simulink model "controladores_LAB4"  (R2023b)
settings: Solver=ode23t  StartTime=0.0  StopTime=110  RelTol=1e-3
values from neighbouring files (symbols this model uses):
  Blo = 8.18575752786119e-06    (= 8.18575752786e-06)    [modeloMATEMATICOFINAL.m]
  Bmo = 2.02156082362446e-07    (= 2.02156082362e-07)    [modeloMATEMATICOFINAL.m]
  CL = double(subs(C_par))    [modeloMATEMATICOFINAL.m]
  DL = double(subs(D_par))    [modeloMATEMATICOFINAL.m]
  do = 0.06862-0.021    (= 0.04762)    [modeloMATEMATICOFINAL.m]
  GL = sysd.a    [modeloMATEMATICOFINAL.m]
  go = 9.81    [modeloMATEMATICOFINAL.m]
  HL = sysd.b    [modeloMATEMATICOFINAL.m]
  Jlo = 0.00100697016255642    (= 0.00100697016256)    [modeloMATEMATICOFINAL.m]
  Jmo = 2.08549279330578e-07    (= 2.08549279331e-07)    [modeloMATEMATICOFINAL.m]
  Kio = 0.00119530882984502    (= 0.00119530882985)    [modeloMATEMATICOFINAL.m]
  Kvo = 0.0035694528924319    (= 0.00356945289243)    [modeloMATEMATICOFINAL.m]
  Lo = 0.667669785204658    (= 0.667669785205)    [modeloMATEMATICOFINAL.m]
  mo = 0.17244    [modeloMATEMATICOFINAL.m]
  no = 120    [modeloMATEMATICOFINAL.m]
  Ro = 5.15610211779038    (= 5.15610211779)    [modeloMATEMATICOFINAL.m]
  Tm = 0.03    [modeloMATEMATICOFINAL.m]
  Vin0 = Ro*X10    (= 0)    [modeloMATEMATICOFINAL.m]
  X10 = 0    [modeloMATEMATICOFINAL.m]
  X20 = 0    [modeloMATEMATICOFINAL.m]
  X30 = 0    [modeloMATEMATICOFINAL.m]
libraries: simulink x8, cstblocks x8
settings Model: Creator=hubertdelgado  LastModifiedBy=automatizacion
settings DebuggingCC: UnconnectedInputMsg=warning  UnconnectedOutputMsg=warning  UnconnectedLineMsg=warning
settings ModelReferenceCC: EnableRefExpFcnMdlSchedulingChecks=on
settings RTWCC: DLArmComputeVersion=19.05

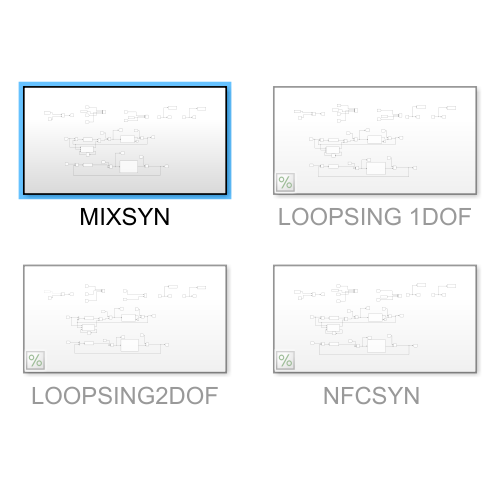
[thumbnail: Simulink's stored preview of the top-level diagram]
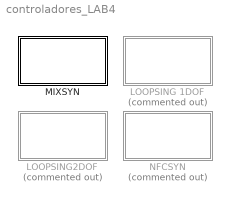
== system controladores_LAB4 ==
  LOOPSING 1DOF : Subsystem  Commented=on
  LOOPSING2DOF : Subsystem  Commented=on
  MIXSYN : Subsystem
  "NFCSYN " : Subsystem  Commented=on

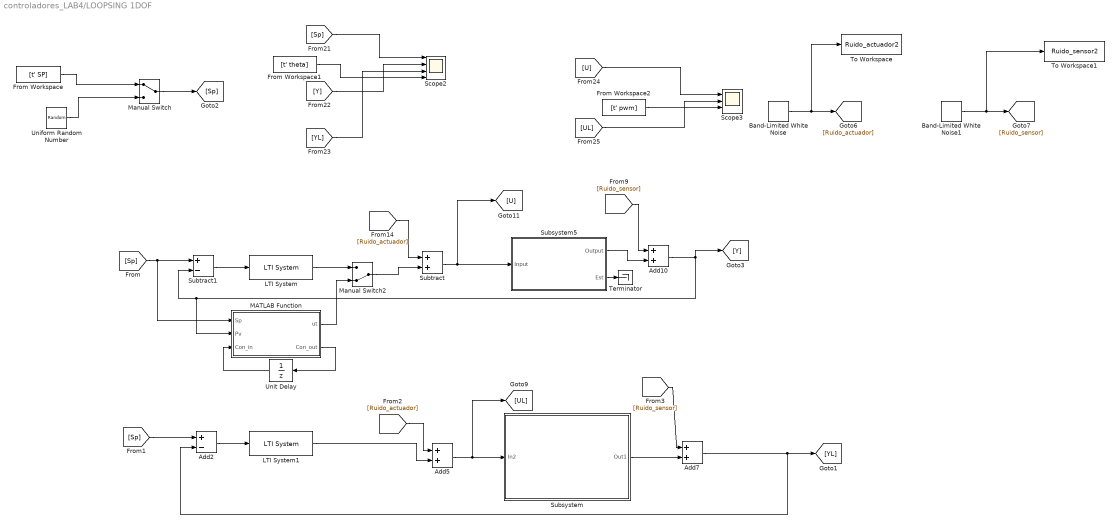
== system controladores_LAB4/LOOPSING 1DOF ==
  Add10 : Sum
  Add2 : Sum  Inputs=+-
  Add5 : Sum
  Add7 : Sum
  Band-Limited White Noise : simulink/Sources/Band-Limited White Noise  Cov=[1e-8]  Ts=0.001  seed=[23341]
  Band-Limited White Noise1 : simulink/Sources/Band-Limited White Noise  Cov=[1e-8]  Ts=0.001  seed=[23341]
  From Workspace : FromWorkspace  VariableName=[t' SP]
  From Workspace1 : FromWorkspace  VariableName=[t' theta]
  From Workspace2 : FromWorkspace  VariableName=[t' pwm]
  LTI System : cstblocks/LTI System  sys=Kred  IC=[]  PadeOrder=0
  LTI System1 : cstblocks/LTI System  sys=Kred  IC=[]  PadeOrder=0
  MATLAB Function : MATLAB Function  TreatAsAtomicUnit=on
  Manual Switch : ManualSwitch
  Manual Switch2 : ManualSwitch  CurrentSetting=0
  Scope2 : Scope  NumInputPorts=4
  Scope3 : Scope  NumInputPorts=3
  Subsystem : Subsystem
  Subsystem5 : Subsystem
  Subtract : Sum
  Subtract1 : Sum  Inputs=+-
  Terminator : Terminator
  To Workspace : ToWorkspace  VariableName=Ruido_actuador2  SampleTime=-1
  To Workspace1 : ToWorkspace  VariableName=Ruido_sensor2  SampleTime=-1
  Uniform Random Number : UniformRandomNumber  Minimum=-70*(pi/180)  Maximum=70*(pi/180)  SampleTime=10
  Unit Delay : UnitDelay  InitialCondition=zeros(4,1)  SampleTime=Tm  HasFrameUpgradeWarning=on
  wires:
  Add5/1 -> [UL], Subsystem/1(In2)
  [Ruido_sensor] -> Add10/1
  [Ruido_actuador] -> Subtract/1
  [Ruido_sensor] -> Add7/1
  Add7/1 -> Add2/2, [YL]
  Subsystem5/1(Output) -> Add10/2
  Subtract/1 -> Subsystem5/1(Input), [U]
  Band-Limited White Noise/1 -> To Workspace/1, [Ruido_actuador]
  Band-Limited White Noise1/1 -> To Workspace1/1, [Ruido_sensor]
  [Ruido_actuador] -> Add5/1
  Add10/1 -> [Y], MATLAB Function/2(Pv), Subtract1/2
  Add2/1 -> LTI System1/1
  [Sp] -> Add2/1
  Subsystem5/2(Est) -> Terminator/1
  Subtract1/1 -> LTI System/1
  LTI System/1 -> Manual Switch2/1
  Manual Switch2/1 -> Subtract/2
  [Sp] -> MATLAB Function/1(Sp), Subtract1/1
  Subsystem/1(Out1) -> Add7/2
  LTI System1/1 -> Add5/2
  Unit Delay/1 -> MATLAB Function/3(Con_in)
  MATLAB Function/1(ut) -> Manual Switch2/2
  MATLAB Function/2(Con_out) -> Unit Delay/1
  [YL] -> Scope2/3
  [Sp] -> Scope2/1
  Uniform Random Number/1 -> Manual Switch/2
  [U] -> Scope3/1
  [UL] -> Scope3/2
  From Workspace/1 -> Manual Switch/1
  Manual Switch/1 -> [Sp]
  [Y] -> Scope2/2
  From Workspace1/1 -> Scope2/4
  From Workspace2/1 -> Scope3/3

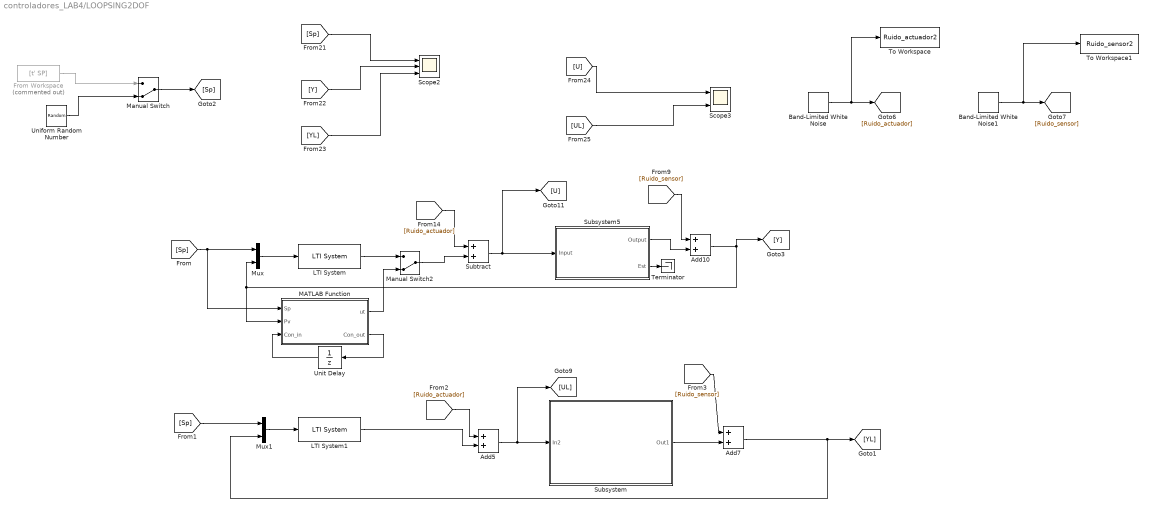
== system controladores_LAB4/LOOPSING2DOF ==
  Add10 : Sum
  Add5 : Sum
  Add7 : Sum
  Band-Limited White Noise : simulink/Sources/Band-Limited White Noise  Cov=[1e-8]  Ts=0.001  seed=[23341]
  Band-Limited White Noise1 : simulink/Sources/Band-Limited White Noise  Cov=[1e-8]  Ts=0.001  seed=[23341]
  From Workspace : FromWorkspace  Commented=on  VariableName=[t' SP]
  LTI System : cstblocks/LTI System  sys=Kred2dof  IC=[]  PadeOrder=0
  LTI System1 : cstblocks/LTI System  sys=Kred2dof  IC=[]  PadeOrder=0
  MATLAB Function : MATLAB Function  TreatAsAtomicUnit=on
  Manual Switch : ManualSwitch  CurrentSetting=0
  Manual Switch2 : ManualSwitch  CurrentSetting=0
  Mux : Mux  Inputs=2
  Mux1 : Mux  Inputs=2
  Scope2 : Scope  NumInputPorts=3
  Scope3 : Scope  NumInputPorts=2
  Subsystem : Subsystem
  Subsystem5 : Subsystem
  Subtract : Sum
  Terminator : Terminator
  To Workspace : ToWorkspace  VariableName=Ruido_actuador2  SampleTime=-1
  To Workspace1 : ToWorkspace  VariableName=Ruido_sensor2  SampleTime=-1
  Uniform Random Number : UniformRandomNumber  Minimum=-70*(pi/180)  Maximum=70*(pi/180)  SampleTime=10
  Unit Delay : UnitDelay  InitialCondition=zeros(5,1)  SampleTime=Tm  HasFrameUpgradeWarning=on
  wires:
  MATLAB Function/1(ut) -> Manual Switch2/2
  Unit Delay/1 -> MATLAB Function/3(Con_in)
  LTI System1/1 -> Add5/2
  Subsystem/1(Out1) -> Add7/2
  [Sp] -> Mux/1, MATLAB Function/1(Sp)
  Manual Switch2/1 -> Subtract/2
  LTI System/1 -> Manual Switch2/1
  Subsystem5/2(Est) -> Terminator/1
  [Sp] -> Mux1/1
  Mux1/1 -> LTI System1/1
  Add10/1 -> Mux/2, MATLAB Function/2(Pv), [Y]
  [Ruido_actuador] -> Add5/1
  Band-Limited White Noise1/1 -> [Ruido_sensor], To Workspace1/1
  Band-Limited White Noise/1 -> [Ruido_actuador], To Workspace/1
  Subtract/1 -> [U], Subsystem5/1(Input)
  Subsystem5/1(Output) -> Add10/2
  Add7/1 -> Mux1/2, [YL]
  [Ruido_sensor] -> Add7/1
  [Ruido_actuador] -> Subtract/1
  [Ruido_sensor] -> Add10/1
  Add5/1 -> Subsystem/1(In2), [UL]
  MATLAB Function/2(Con_out) -> Unit Delay/1
  Mux/1 -> LTI System/1
  [Y] -> Scope2/2
  [U] -> Scope3/1
  From Workspace/1 -> Manual Switch/1
  Uniform Random Number/1 -> Manual Switch/2
  [UL] -> Scope3/2
  [YL] -> Scope2/3
  [Sp] -> Scope2/1
  Manual Switch/1 -> [Sp]

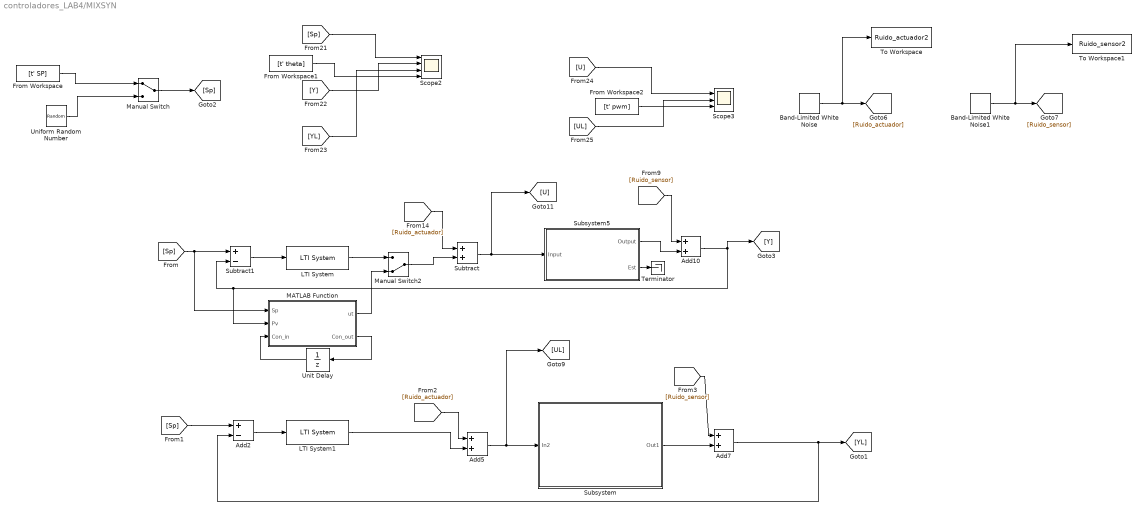
== system controladores_LAB4/MIXSYN ==
  Add10 : Sum
  Add2 : Sum  Inputs=+-
  Add5 : Sum
  Add7 : Sum
  Band-Limited White Noise : simulink/Sources/Band-Limited White Noise  Cov=[1e-8]  Ts=0.001  seed=[23341]
  Band-Limited White Noise1 : simulink/Sources/Band-Limited White Noise  Cov=[1e-8]  Ts=0.001  seed=[23341]
  From Workspace : FromWorkspace  VariableName=[t' SP]
  From Workspace1 : FromWorkspace  VariableName=[t' theta]
  From Workspace2 : FromWorkspace  VariableName=[t' pwm]
  LTI System : cstblocks/LTI System  sys=Kred  IC=[]  PadeOrder=0
  LTI System1 : cstblocks/LTI System  sys=Kred  IC=[]  PadeOrder=0
  MATLAB Function : MATLAB Function  TreatAsAtomicUnit=on
  Manual Switch : ManualSwitch
  Manual Switch2 : ManualSwitch  CurrentSetting=0
  Scope2 : Scope  NumInputPorts=4
  Scope3 : Scope  NumInputPorts=3
  Subsystem : Subsystem
  Subsystem5 : Subsystem
  Subtract : Sum
  Subtract1 : Sum  Inputs=+-
  Terminator : Terminator
  To Workspace : ToWorkspace  VariableName=Ruido_actuador2  SampleTime=-1
  To Workspace1 : ToWorkspace  VariableName=Ruido_sensor2  SampleTime=-1
  Uniform Random Number : UniformRandomNumber  Minimum=-70*(pi/180)  Maximum=70*(pi/180)  SampleTime=10
  Unit Delay : UnitDelay  InitialCondition=zeros(5,1)  SampleTime=Tm  HasFrameUpgradeWarning=on
  wires:
  [Sp] -> Scope2/1
  Add5/1 -> [UL], Subsystem/1(In2)
  [Ruido_sensor] -> Add10/1
  [Ruido_actuador] -> Subtract/1
  [Ruido_sensor] -> Add7/1
  Add7/1 -> Add2/2, [YL]
  [Y] -> Scope2/2
  Subsystem5/1(Output) -> Add10/2
  [YL] -> Scope2/3
  Subtract/1 -> Subsystem5/1(Input), [U]
  Band-Limited White Noise/1 -> To Workspace/1, [Ruido_actuador]
  Band-Limited White Noise1/1 -> To Workspace1/1, [Ruido_sensor]
  Manual Switch/1 -> [Sp]
  [UL] -> Scope3/2
  From Workspace/1 -> Manual Switch/1
  [U] -> Scope3/1
  Uniform Random Number/1 -> Manual Switch/2
  [Ruido_actuador] -> Add5/1
  Add10/1 -> [Y], MATLAB Function/2(Pv), Subtract1/2
  Add2/1 -> LTI System1/1
  [Sp] -> Add2/1
  Subsystem5/2(Est) -> Terminator/1
  Subtract1/1 -> LTI System/1
  LTI System/1 -> Manual Switch2/1
  Manual Switch2/1 -> Subtract/2
  [Sp] -> MATLAB Function/1(Sp), Subtract1/1
  Subsystem/1(Out1) -> Add7/2
  LTI System1/1 -> Add5/2
  Unit Delay/1 -> MATLAB Function/3(Con_in)
  MATLAB Function/1(ut) -> Manual Switch2/2
  MATLAB Function/2(Con_out) -> Unit Delay/1
  From Workspace1/1 -> Scope2/4
  From Workspace2/1 -> Scope3/3

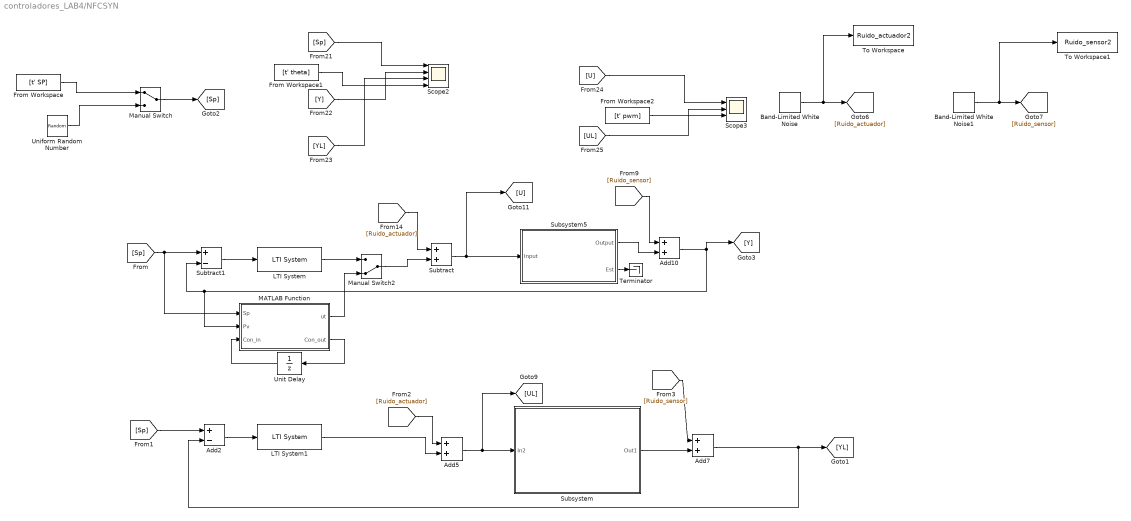
== system controladores_LAB4/NFCSYN  ==
  Add10 : Sum
  Add2 : Sum  Inputs=+-
  Add5 : Sum
  Add7 : Sum
  Band-Limited White Noise : simulink/Sources/Band-Limited White Noise  Cov=[1e-8]  Ts=0.001  seed=[23341]
  Band-Limited White Noise1 : simulink/Sources/Band-Limited White Noise  Cov=[1e-8]  Ts=0.001  seed=[23341]
  From Workspace : FromWorkspace  VariableName=[t' SP]
  From Workspace1 : FromWorkspace  VariableName=[t' theta]
  From Workspace2 : FromWorkspace  VariableName=[t' pwm]
  LTI System : cstblocks/LTI System  sys=Kred  IC=[]  PadeOrder=0
  LTI System1 : cstblocks/LTI System  sys=Kred  IC=[]  PadeOrder=0
  MATLAB Function : MATLAB Function  TreatAsAtomicUnit=on
  Manual Switch : ManualSwitch
  Manual Switch2 : ManualSwitch  CurrentSetting=0
  Scope2 : Scope  NumInputPorts=4
  Scope3 : Scope  NumInputPorts=3
  Subsystem : Subsystem
  Subsystem5 : Subsystem
  Subtract : Sum
  Subtract1 : Sum  Inputs=+-
  Terminator : Terminator
  To Workspace : ToWorkspace  VariableName=Ruido_actuador2  SampleTime=-1
  To Workspace1 : ToWorkspace  VariableName=Ruido_sensor2  SampleTime=-1
  Uniform Random Number : UniformRandomNumber  Minimum=-70*(pi/180)  Maximum=70*(pi/180)  SampleTime=10
  Unit Delay : UnitDelay  InitialCondition=zeros(4,1)  SampleTime=Tm  HasFrameUpgradeWarning=on
  wires:
  Add5/1 -> [UL], Subsystem/1(In2)
  [Ruido_sensor] -> Add10/1
  [Ruido_actuador] -> Subtract/1
  [Ruido_sensor] -> Add7/1
  Add7/1 -> Add2/2, [YL]
  Subsystem5/1(Output) -> Add10/2
  Subtract/1 -> Subsystem5/1(Input), [U]
  Band-Limited White Noise/1 -> To Workspace/1, [Ruido_actuador]
  Band-Limited White Noise1/1 -> To Workspace1/1, [Ruido_sensor]
  [Ruido_actuador] -> Add5/1
  Add10/1 -> [Y], MATLAB Function/2(Pv), Subtract1/2
  Add2/1 -> LTI System1/1
  [Sp] -> Add2/1
  Subsystem5/2(Est) -> Terminator/1
  Subtract1/1 -> LTI System/1
  LTI System/1 -> Manual Switch2/1
  Manual Switch2/1 -> Subtract/2
  [Sp] -> MATLAB Function/1(Sp), Subtract1/1
  Subsystem/1(Out1) -> Add7/2
  LTI System1/1 -> Add5/2
  Unit Delay/1 -> MATLAB Function/3(Con_in)
  MATLAB Function/1(ut) -> Manual Switch2/2
  MATLAB Function/2(Con_out) -> Unit Delay/1
  From Workspace1/1 -> Scope2/4
  [Y] -> Scope2/2
  [U] -> Scope3/1
  From Workspace/1 -> Manual Switch/1
  Uniform Random Number/1 -> Manual Switch/2
  [UL] -> Scope3/2
  [YL] -> Scope2/3
  [Sp] -> Scope2/1
  Manual Switch/1 -> [Sp]
  From Workspace2/1 -> Scope3/3

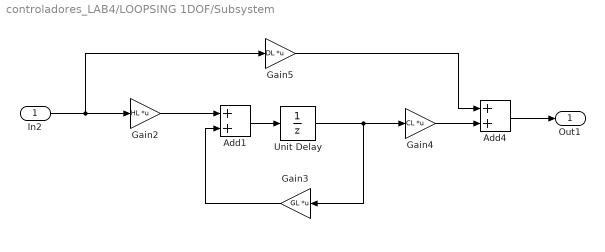
== system controladores_LAB4/LOOPSING 1DOF/Subsystem ==
  In2 : Inport
  Add1 : Sum
  Add4 : Sum
  Gain2 : Gain  Gain=HL  Multiplication=Matrix(K*u)
  Gain3 : Gain  Gain=GL  Multiplication=Matrix(K*u)
  Gain4 : Gain  Gain=CL  Multiplication=Matrix(K*u)
  Gain5 : Gain  Gain=DL  Multiplication=Matrix(K*u)
  Unit Delay : UnitDelay  SampleTime=Tm  HasFrameUpgradeWarning=on
  Out1 : Outport
  wires:
  Add4/1 -> Out1/1
  Gain4/1 -> Add4/2
  Gain3/1 -> Add1/2
  Add1/1 -> Unit Delay/1
  In2/1 -> Gain5/1, Gain2/1
  Unit Delay/1 -> Gain4/1, Gain3/1
  Gain2/1 -> Add1/1
  Gain5/1 -> Add4/1

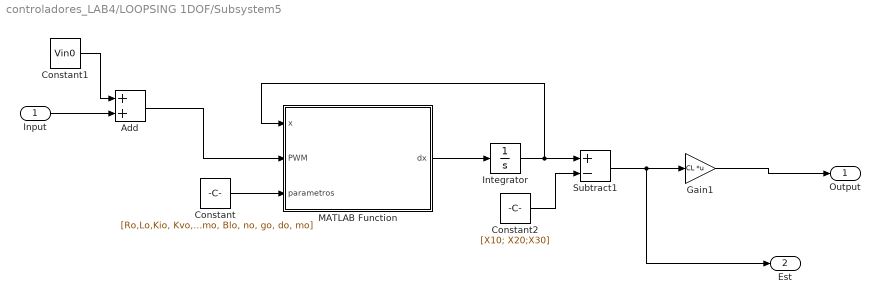
== system controladores_LAB4/LOOPSING 1DOF/Subsystem5 ==
  Input : Inport
  Add : Sum
  Constant : Constant  Value=[Ro,Lo,Kio, Kvo, Jmo, Jlo, Bmo, Blo, no, go, do, mo]
  Constant1 : Constant  Value=Vin0
  Constant2 : Constant  Value=[X10; X20;X30]
  Gain1 : Gain  Gain=CL  Multiplication=Matrix(K*u)
  Integrator : Integrator  InitialCondition=[X10; X20;X30]
  MATLAB Function : MATLAB Function  TreatAsAtomicUnit=on
  Subtract1 : Sum  Inputs=+-
  Output : Outport
  Est : Outport  Port=2
  wires:
  Add/1 -> MATLAB Function/2(PWM)
  Constant2/1 -> Subtract1/2
  Constant1/1 -> Add/1
  Input/1 -> Add/2
  MATLAB Function/1(dx) -> Integrator/1
  Constant/1 -> MATLAB Function/3(parametros)
  Integrator/1 -> Subtract1/1, MATLAB Function/1(x)
  Subtract1/1 -> Est/1, Gain1/1
  Gain1/1 -> Output/1

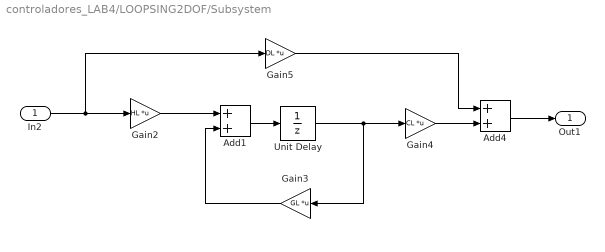
== system controladores_LAB4/LOOPSING2DOF/Subsystem ==
  In2 : Inport
  Add1 : Sum
  Add4 : Sum
  Gain2 : Gain  Gain=HL  Multiplication=Matrix(K*u)
  Gain3 : Gain  Gain=GL  Multiplication=Matrix(K*u)
  Gain4 : Gain  Gain=CL  Multiplication=Matrix(K*u)
  Gain5 : Gain  Gain=DL  Multiplication=Matrix(K*u)
  Unit Delay : UnitDelay  SampleTime=Tm  HasFrameUpgradeWarning=on
  Out1 : Outport
  wires:
  Gain5/1 -> Add4/1
  Gain2/1 -> Add1/1
  Unit Delay/1 -> Gain3/1, Gain4/1
  In2/1 -> Gain2/1, Gain5/1
  Add1/1 -> Unit Delay/1
  Gain3/1 -> Add1/2
  Gain4/1 -> Add4/2
  Add4/1 -> Out1/1

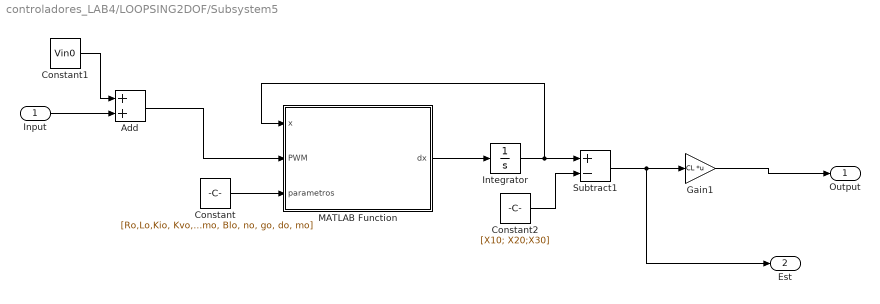
== system controladores_LAB4/LOOPSING2DOF/Subsystem5 ==
  Input : Inport
  Add : Sum
  Constant : Constant  Value=[Ro,Lo,Kio, Kvo, Jmo, Jlo, Bmo, Blo, no, go, do, mo]
  Constant1 : Constant  Value=Vin0
  Constant2 : Constant  Value=[X10; X20;X30]
  Gain1 : Gain  Gain=CL  Multiplication=Matrix(K*u)
  Integrator : Integrator  InitialCondition=[X10; X20;X30]
  MATLAB Function : MATLAB Function  TreatAsAtomicUnit=on
  Subtract1 : Sum  Inputs=+-
  Output : Outport
  Est : Outport  Port=2
  wires:
  Gain1/1 -> Output/1
  Subtract1/1 -> Gain1/1, Est/1
  Integrator/1 -> MATLAB Function/1(x), Subtract1/1
  Constant/1 -> MATLAB Function/3(parametros)
  MATLAB Function/1(dx) -> Integrator/1
  Input/1 -> Add/2
  Constant1/1 -> Add/1
  Constant2/1 -> Subtract1/2
  Add/1 -> MATLAB Function/2(PWM)

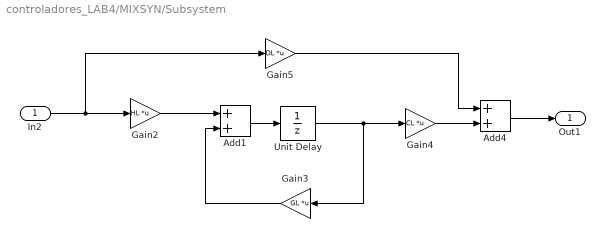
== system controladores_LAB4/MIXSYN/Subsystem ==
  In2 : Inport
  Add1 : Sum
  Add4 : Sum
  Gain2 : Gain  Gain=HL  Multiplication=Matrix(K*u)
  Gain3 : Gain  Gain=GL  Multiplication=Matrix(K*u)
  Gain4 : Gain  Gain=CL  Multiplication=Matrix(K*u)
  Gain5 : Gain  Gain=DL  Multiplication=Matrix(K*u)
  Unit Delay : UnitDelay  SampleTime=Tm  HasFrameUpgradeWarning=on
  Out1 : Outport
  wires:
  Add4/1 -> Out1/1
  Gain4/1 -> Add4/2
  Gain3/1 -> Add1/2
  Add1/1 -> Unit Delay/1
  In2/1 -> Gain5/1, Gain2/1
  Unit Delay/1 -> Gain4/1, Gain3/1
  Gain2/1 -> Add1/1
  Gain5/1 -> Add4/1

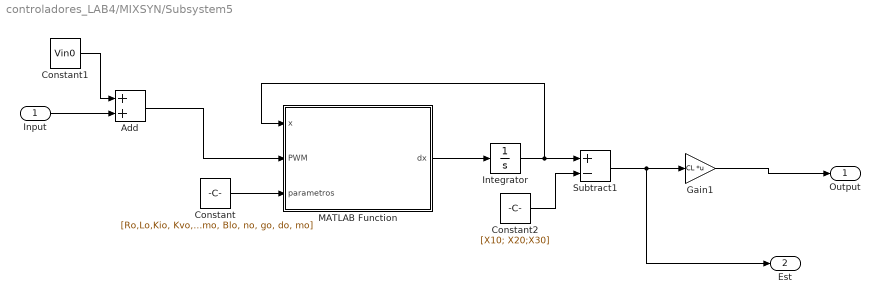
== system controladores_LAB4/MIXSYN/Subsystem5 ==
  Input : Inport
  Add : Sum
  Constant : Constant  Value=[Ro,Lo,Kio, Kvo, Jmo, Jlo, Bmo, Blo, no, go, do, mo]
  Constant1 : Constant  Value=Vin0
  Constant2 : Constant  Value=[X10; X20;X30]
  Gain1 : Gain  Gain=CL  Multiplication=Matrix(K*u)
  Integrator : Integrator  InitialCondition=[X10; X20;X30]
  MATLAB Function : MATLAB Function  TreatAsAtomicUnit=on
  Subtract1 : Sum  Inputs=+-
  Output : Outport
  Est : Outport  Port=2
  wires:
  Add/1 -> MATLAB Function/2(PWM)
  Constant2/1 -> Subtract1/2
  Constant1/1 -> Add/1
  Input/1 -> Add/2
  MATLAB Function/1(dx) -> Integrator/1
  Constant/1 -> MATLAB Function/3(parametros)
  Integrator/1 -> Subtract1/1, MATLAB Function/1(x)
  Subtract1/1 -> Est/1, Gain1/1
  Gain1/1 -> Output/1

== system controladores_LAB4/NFCSYN /Subsystem ==
  In2 : Inport
  Add1 : Sum
  Add4 : Sum
  Gain2 : Gain  Gain=HL  Multiplication=Matrix(K*u)
  Gain3 : Gain  Gain=GL  Multiplication=Matrix(K*u)
  Gain4 : Gain  Gain=CL  Multiplication=Matrix(K*u)
  Gain5 : Gain  Gain=DL  Multiplication=Matrix(K*u)
  Unit Delay : UnitDelay  SampleTime=Tm  HasFrameUpgradeWarning=on
  Out1 : Outport
  wires:
  Add4/1 -> Out1/1
  Gain4/1 -> Add4/2
  Gain3/1 -> Add1/2
  Add1/1 -> Unit Delay/1
  In2/1 -> Gain5/1, Gain2/1
  Unit Delay/1 -> Gain4/1, Gain3/1
  Gain2/1 -> Add1/1
  Gain5/1 -> Add4/1

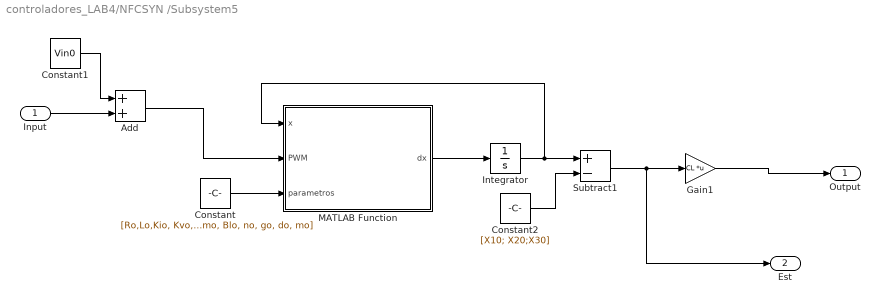
== system controladores_LAB4/NFCSYN /Subsystem5 ==
  Input : Inport
  Add : Sum
  Constant : Constant  Value=[Ro,Lo,Kio, Kvo, Jmo, Jlo, Bmo, Blo, no, go, do, mo]
  Constant1 : Constant  Value=Vin0
  Constant2 : Constant  Value=[X10; X20;X30]
  Gain1 : Gain  Gain=CL  Multiplication=Matrix(K*u)
  Integrator : Integrator  InitialCondition=[X10; X20;X30]
  MATLAB Function : MATLAB Function  TreatAsAtomicUnit=on
  Subtract1 : Sum  Inputs=+-
  Output : Outport
  Est : Outport  Port=2
  wires:
  Add/1 -> MATLAB Function/2(PWM)
  Constant2/1 -> Subtract1/2
  Constant1/1 -> Add/1
  Input/1 -> Add/2
  MATLAB Function/1(dx) -> Integrator/1
  Constant/1 -> MATLAB Function/3(parametros)
  Integrator/1 -> Subtract1/1, MATLAB Function/1(x)
  Subtract1/1 -> Est/1, Gain1/1
  Gain1/1 -> Output/1

== matlab function controladores_LAB4/MIXSYN/MATLAB Function ==
  data: Sp input; ut output; Pv input; Con_in input; Con_out output
function [ut, Con_out] = fcn(Sp,Pv,Con_in)

xk = Con_in(1:4); % Estados controlador
Du = Con_in(5); % Actuadores
% Diseño mixsyn
Gc = [0.999707105424673,0.00151771236953691,0.000689904726261718,-0.000339220737457422;-0.00151772398850250,0.756753569411887,-0.321971210474965,0.0952642884793470;0.000689878641928251,0.321971196611839,0.627937488408591,0.244883619731361;-0.000339193385452838,-0.0952642611575348,0.244883581403790,0.768717841221103];
Hc = [13.3897425159846;34.4454472814104;-15.9073661414958;7.78030172576614];
Cc = [0.100423050184375,-0.258340858953882,-0.119305245563825,0.0583522705240672];
Dc = [34.7870470020576];

Ka = zeros(1,1); 

Sp = [Sp];
Pv = [Pv];
error = Sp-Pv;
xk_1 = Gc*xk+Hc*error - Ka*Du;
u = Cc*xk+Dc*error;


u1s = u; 

if u>=100
    u1s = 100;
end
if u<=-100
    u1s = -100;
end

Du = u - u1s;
ut = u1s;

Con_out = [xk_1; Du];

== matlab function controladores_LAB4/LOOPSING 1DOF/MATLAB Function ==
  data: Sp input; ut output; Pv input; Con_in input; Con_out output
function [ut, Con_out] = fcn(Sp,Pv,Con_in)

xk = Con_in(1:3); % Estados controlador
Du = Con_in(4); % Actuadores

% Diseño loopsyn
Gc = [0.385387352026787	-0.351868912104334	0
0.351868912104333	0.104011862141422	0
0	0	1];
Hc = [73.4809041059298
-11.4856211615732
-293.409177798269];
Cc = [-0.551106780794473	-0.0861421587117992	-0.00390881653780578];
Dc = [64.540387713901720];


Ka = zeros(1,1); 

Sp = [Sp];
Pv = [Pv];
error = Sp-Pv;
xk_1 = Gc*xk+Hc*error - Ka*Du;
u = Cc*xk+Dc*error;


u1s = u; 

if u>=100
    u1s = 100;
end
if u<=-100
    u1s = -100;
end

Du = u - u1s;
ut = u1s;

Con_out = [xk_1; Du];

== matlab function controladores_LAB4/LOOPSING 1DOF/Subsystem5/MATLAB Function ==
  data: x input; PWM input; dx output; parametros input
function dx = fcn(x,PWM,parametros)

%ESTADOS
x1 = x(1);
x2 = x(2);
x3 = x(3);

%Parametros
R = parametros(1);
L = parametros(2);
Ki = parametros(3);
Kv = parametros(4);
Jm = parametros(5);
Jl = parametros(6);
Bm = parametros(7);
Bl = parametros(8);
n = parametros(9);
g = parametros(10);
d = parametros(11);
m = parametros(12);

%EXPRESIONES
% Jt = Jm*n^2 +Jl;
% f1 = (1/L)*(((7*PWM)/100) - R*x1 - Kv*x2*n);
% f2 = (1/Jt)*(Ki*x1*n - (Bm*n^2 + Bl)*x2 - m*g*d*sin(x3));
% f3 = x2;

% MODELO 2 ESTADOS I TL WL  SALIDA TL WL
f1 = (((7*PWM)/100)-Kv*x3*n-R*x1)/(L); %di/dt
f2 = x3; %d0l/dt = Wl
f3 = ((Ki*x1*n)-x3*(Bm*n^2+Bl)-(m*g*d*sin(x2)))/(Jl+Jm*n^2);  %dwl/dt 

dx = [f1; f2; f3];

== matlab function controladores_LAB4/LOOPSING2DOF/MATLAB Function ==
  data: Sp input; ut output; Pv input; Con_in input; Con_out output
function [ut, Con_out] = fcn(Sp,Pv,Con_in)

xk = Con_in(1:4); % Estados controlador
Du = Con_in(5); % Actuadores

% Diseño loopsyn 2DOF
Gc = [0.387740952147887	-0.330773217755832	0.0933023055793410	0
0.302858443809632	0.398806974639918	0.531579394339184	0
-0.122147507991330	0.367784789347473	0.241457501845062	0
0	0	0	1];
Hc = [ 7.49504652749455	-73.3356874631247
-9.61892940173992	7.89345204191609
-9.64896526640991	-6.79243127064359
-293.409177798267	293.409177798269];
Cc = [-0.553683399270205	-0.0742928123337326	0.0396733540563608	-0.00390881653780578];
Dc = [32.7641447476837	-64.5403877139017];

Ka = zeros(1,1); 

xk_1 = Gc*xk + Hc*[Sp; Pv] - Ka*Du;
u = Cc*xk + Dc*[Sp; Pv];

u1s = u; 

if u>=100
    u1s = 100;
end
if u<=-100
    u1s = -100;
end

Du = u - u1s;
ut = u1s;

Con_out = [xk_1; Du];

== matlab function controladores_LAB4/LOOPSING2DOF/Subsystem5/MATLAB Function ==
  data: x input; PWM input; dx output; parametros input
function dx = fcn(x,PWM,parametros)

%ESTADOS
x1 = x(1);
x2 = x(2);
x3 = x(3);

%Parametros
R = parametros(1);
L = parametros(2);
Ki = parametros(3);
Kv = parametros(4);
Jm = parametros(5);
Jl = parametros(6);
Bm = parametros(7);
Bl = parametros(8);
n = parametros(9);
g = parametros(10);
d = parametros(11);
m = parametros(12);

%EXPRESIONES
% Jt = Jm*n^2 +Jl;
% f1 = (1/L)*(((7*PWM)/100) - R*x1 - Kv*x2*n);
% f2 = (1/Jt)*(Ki*x1*n - (Bm*n^2 + Bl)*x2 - m*g*d*sin(x3));
% f3 = x2;

% MODELO 2 ESTADOS I TL WL  SALIDA TL WL
f1 = (((7*PWM)/100)-Kv*x3*n-R*x1)/(L); %di/dt
f2 = x3; %d0l/dt = Wl
f3 = ((Ki*x1*n)-x3*(Bm*n^2+Bl)-(m*g*d*sin(x2)))/(Jl+Jm*n^2);  %dwl/dt 

dx = [f1; f2; f3];

== matlab function controladores_LAB4/NFCSYN /MATLAB Function ==
  data: Sp input; ut output; Pv input; Con_in input; Con_out output
function [ut, Con_out] = fcn(Sp,Pv,Con_in)

xk = Con_in(1:3); % Estados controlador
Du = Con_in(4); % Actuadores

% Diseño nfcsyn
Gc = [0.853862925588747	0.187830959530800	0
-0.187830959530800	0.954205726727783	0
0	0	1];
Hc = [-8.29512388959399
-1.99815784321956
-101.934103302858];
Cc = [-0.0622134291719549	0.0149861838241466	-0.00900000000000000];
Dc = [0];


Ka = zeros(1,1); 

Sp = [Sp];
Pv = [Pv];
error = Sp-Pv;
xk_1 = Gc*xk+Hc*error - Ka*Du;
u = Cc*xk+Dc*error;


u1s = u; 

if u>=100
    u1s = 100;
end
if u<=-100
    u1s = -100;
end

Du = u - u1s;
ut = u1s;

Con_out = [xk_1; Du];

== matlab function controladores_LAB4/NFCSYN /Subsystem5/MATLAB Function ==
  data: x input; PWM input; dx output; parametros input
function dx = fcn(x,PWM,parametros)

%ESTADOS
x1 = x(1);
x2 = x(2);
x3 = x(3);

%Parametros
R = parametros(1);
L = parametros(2);
Ki = parametros(3);
Kv = parametros(4);
Jm = parametros(5);
Jl = parametros(6);
Bm = parametros(7);
Bl = parametros(8);
n = parametros(9);
g = parametros(10);
d = parametros(11);
m = parametros(12);

%EXPRESIONES
% Jt = Jm*n^2 +Jl;
% f1 = (1/L)*(((7*PWM)/100) - R*x1 - Kv*x2*n);
% f2 = (1/Jt)*(Ki*x1*n - (Bm*n^2 + Bl)*x2 - m*g*d*sin(x3));
% f3 = x2;

% MODELO 2 ESTADOS I TL WL  SALIDA TL WL
f1 = (((7*PWM)/100)-Kv*x3*n-R*x1)/(L); %di/dt
f2 = x3; %d0l/dt = Wl
f3 = ((Ki*x1*n)-x3*(Bm*n^2+Bl)-(m*g*d*sin(x2)))/(Jl+Jm*n^2);  %dwl/dt 

dx = [f1; f2; f3];

== matlab function controladores_LAB4/MIXSYN/Subsystem5/MATLAB Function ==
  data: x input; PWM input; dx output; parametros input
function dx = fcn(x,PWM,parametros)

%ESTADOS
x1 = x(1);
x2 = x(2);
x3 = x(3);

%Parametros
R = parametros(1);
L = parametros(2);
Ki = parametros(3);
Kv = parametros(4);
Jm = parametros(5);
Jl = parametros(6);
Bm = parametros(7);
Bl = parametros(8);
n = parametros(9);
g = parametros(10);
d = parametros(11);
m = parametros(12);

%EXPRESIONES
% Jt = Jm*n^2 +Jl;
% f1 = (1/L)*(((7*PWM)/100) - R*x1 - Kv*x2*n);
% f2 = (1/Jt)*(Ki*x1*n - (Bm*n^2 + Bl)*x2 - m*g*d*sin(x3));
% f3 = x2;

% MODELO 2 ESTADOS I TL WL  SALIDA TL WL
f1 = (((7*PWM)/100)-Kv*x3*n-R*x1)/(L); %di/dt
f2 = x3; %d0l/dt = Wl
f3 = ((Ki*x1*n)-x3*(Bm*n^2+Bl)-(m*g*d*sin(x2)))/(Jl+Jm*n^2);  %dwl/dt 

dx = [f1; f2; f3];
